simulink model "gm_HDLAWGNGenerator"  (R2021a)
settings: Solver=FixedStepDiscrete  StartTime=0.0  StopTime=StopTime  RelTol=1e-3
InitFcn:
  | whdlexamples.hdlawgn_init
undefined symbols (not defined in the file or in its folder): coefficientsSqrt1, coefficientsSqrt2, SamplingTime, seedsURNG1, seedsURNG2
libraries: hdlsllib x22, simulink x21, dspsrcs4 x1
(part 2 of 2)

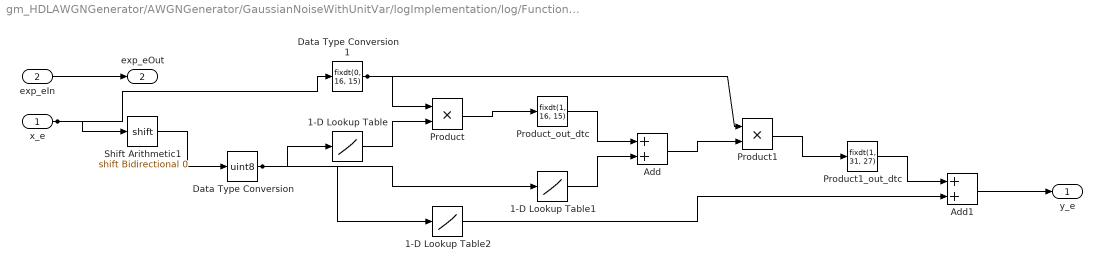
== system gm_HDLAWGNGenerator/AWGNGenerator/GaussianNoiseWithUnitVar/logImplementation/log/FunctionEvaluation ==
  x_e : Inport  OutDataTypeStr=fixdt(0, 49, 48)  PortDimensions=1  SampleTime=1e-06
  exp_eIn : Inport  Port=2  OutDataTypeStr=uint8  PortDimensions=1  SampleTime=1e-06
  1-D Lookup Table : Lookup_n-D  NumberOfTableDimensions=1  BreakpointsForDimension1="fi(\"numerictype\",numerictype(0,8,0),\"fimath\",fimath(\"RoundingMethod\", \"Nearest\",\"OverflowAction\", \"Saturate\",\"ProductMode\",\"FullPrecision\",\"SumMode\",\"FullPrecision\"),\"Value\",\"[0 1 2 3 4 5 6 7 8 9 10 11 12 13 14 15 16 17 18 19 20 21 22 23 24 25 26 27 28 29 30 31 32 33 34 35 36 37 38 39 40 41 42 43 44 45 46 47 48 49 50 51 52 53 54 55 56 57 58 59 60 61 62 63 64 65 66 67 68 69 70 71 72 73 74 75 76 77 78 79 80 81 82 83 84 85 86 87 88 89 90 91 92 93 94 95 96 97 98 99 100 101 102 103 104 105 106 107 108 109 110 111 112 113 114 115 116 117 118 119 120 121 122 123 124 125 126 127 128 129 130 131 132 133 134 135 136 137 138 139 140 141 142 143 144 145 146 147 148 149 150 151 152 153 154 155 156 157 158 159 160 161 162 163 164 165 166 167 168 169 170 171 172 173 174 175 176 177 178 179 180 181 182 183 184 185 186 187 188 189 190 191 192 193 194 195 196 197 198 199 200 201 202 203 204 205 206 207 208 209 210 211 212 213 214 215 216 217 218 219 220 221 222 223 224 225 226 227 228 229 230 231 232 233 234 235 236 237 238 239 240 241 242 243 244 245 246 247 248 249 250 251 252 253 254 255]\")"  Table="reshape(fi(\"numerictype\",numerictype(1,16,15),\"fimath\",fimath(\"RoundingMethod\", \"Floor\",\"OverflowAction\", \"Wrap\",\"ProductMode\",\"FullPrecision\",\"SumMode\",\"FullPrecision\"),\"Value\",\"[-0.498046875;-0.49420166015625;-0.490386962890625;-0.486602783203125;-0.482879638671875;-0.47918701171875;-0.475555419921875;-0.471954345703125;-0.4683837890625;-0.464874267578125;-0.46136474609375;-0.45794677734375;-0.45452880859375;-0.451171875;-0.447845458984375;-0.444549560546875;-0.4412841796875;-0.43804931640625;-0.43487548828125;-0.431732177734375;-0.428619384765625;-0.425537109375;-0.4224853515625;-0.419464111328125;-0.416473388671875;-0.41351318359375;-0.41058349609375;-0.40771484375;-0.40484619140625;-0.402008056640625;-0.399200439453125;-0.39642333984375;-0.393707275390625;-0.3909912109375;-0.3883056640625;-0.3856201171875;-0.38299560546875;-0.380401611328125;-0.3778076171875;-0.375274658203125;-0.37274169921875;-0.3702392578125;-0.367767333984375;-0.36529541015625;-0.362884521484375;-0.3604736328125;-0.35809326171875;-0.355743408203125;-0.3533935546875;-0.351104736328125;-0.34881591796875;-0.3465576171875;-0.34429931640625;-0.342071533203125;-0.339874267578125;-0.33770751953125;-0.335540771484375;-0.333404541015625;-0.331298828125;-0.329193115234375;-0.327117919921875;-0.3250732421875;-0.323028564453125;-0.321014404296875;-0.319000244140625;-0.3170166015625;-0.3150634765625;-0.3131103515625;-0.311187744140625;-0.30926513671875;-0.307373046875;-0.305511474609375;-0.30364990234375;-0.30181884765625;-0.29998779296875;-0.298187255859375;-0.29638671875;-0.29461669921875;-0.2928466796875;-0.291107177734375;-0.289398193359375;-0.287689208984375;-0.285980224609375;-0.2843017578125;-0.282623291015625;-0.280975341796875;-0.279327392578125;-0.2777099609375;-0.276092529296875;-0.274505615234375;-0.272918701171875;-0.2713623046875;-0.269805908203125;-0.26824951171875;-0.2667236328125;-0.265228271484375;-0.263702392578125;-0.262237548828125;-0.2607421875;-0.25927734375;-0.257843017578125;-0.256378173828125;-0.254974365234375;-0.2535400390625;-0.25213623046875;-0.250732421875;-0.249359130859375;-0.24798583984375;-0.24664306640625;-0.24530029296875;-0.24395751953125;-0.24261474609375;-0.241302490234375;-0.240020751953125;-0.23870849609375;-0.2374267578125;-0.23614501953125;-0.234893798828125;-0.233642578125;-0.232391357421875;-0.231170654296875;-0.229949951171875;-0.228729248046875;-0.227508544921875;-0.226318359375;-0.22515869140625;-0.223968505859375;-0.222808837890625;-0.221649169921875;-0.220489501953125;-0.2193603515625;-0.218231201171875;-0.21710205078125;-0.21600341796875;-0.214874267578125;-0.213775634765625;-0.21270751953125;-0.21160888671875;-0.210540771484375;-0.20947265625;-0.20843505859375;-0.2073974609375;-0.20635986328125;-0.205322265625;-0.20428466796875;-0.203277587890625;-0.2022705078125;-0.201263427734375;-0.20025634765625;-0.19927978515625;-0.19830322265625;-0.19732666015625;-0.196380615234375;-0.195404052734375;-0.1944580078125;-0.193511962890625;-0.19256591796875;-0.191650390625;-0.19073486328125;-0.1898193359375;-0.18890380859375;-0.18798828125;-0.187103271484375;-0.186187744140625;-0.185333251953125;-0.1844482421875;-0.183563232421875;-0.182708740234375;-0.181854248046875;-0.180999755859375;-0.180145263671875;-0.179290771484375;-0.178466796875;-0.177642822265625;-0.17681884765625;-0.175994873046875;-0.1751708984375;-0.17437744140625;-0.173553466796875;-0.172760009765625;-0.171966552734375;-0.17120361328125;-0.17041015625;-0.169647216796875;-0.16888427734375;-0.168121337890625;-0.1673583984375;-0.166595458984375;-0.16583251953125;-0.16510009765625;-0.16436767578125;-0.16363525390625;-0.16290283203125;-0.16217041015625;-0.161468505859375;-0.160736083984375;-0.1600341796875;-0.159332275390625;-0.15863037109375;-0.157928466796875;-0.157257080078125;-0.15655517578125;-0.1558837890625;-0.155181884765625;-0.154510498046875;-0.153839111328125;-0.1531982421875;-0.15252685546875;-0.151885986328125;-0.151214599609375;-0.15057373046875;-0.149932861328125;-0.1492919921875;-0.148651123046875;-0.14801025390625;-0.14739990234375;-0.146759033203125;-0.146148681640625;-0.145538330078125;-0.144927978515625 ...(+656 chars)]\"), [256    1])"  InterpMethod=Flat  ExtrapMethod=Clip  DiagnosticForOutOfRangeInput=Error  SampleTime=1e-06  OutDataTypeStr=fixdt(1, 16, 15)  RndMeth=Simplest  InputSameDT=on
  1-D Lookup Table1 : Lookup_n-D  NumberOfTableDimensions=1  BreakpointsForDimension1="fi(\"numerictype\",numerictype(0,8,0),\"fimath\",fimath(\"RoundingMethod\", \"Nearest\",\"OverflowAction\", \"Saturate\",\"ProductMode\",\"FullPrecision\",\"SumMode\",\"FullPrecision\"),\"Value\",\"[0 1 2 3 4 5 6 7 8 9 10 11 12 13 14 15 16 17 18 19 20 21 22 23 24 25 26 27 28 29 30 31 32 33 34 35 36 37 38 39 40 41 42 43 44 45 46 47 48 49 50 51 52 53 54 55 56 57 58 59 60 61 62 63 64 65 66 67 68 69 70 71 72 73 74 75 76 77 78 79 80 81 82 83 84 85 86 87 88 89 90 91 92 93 94 95 96 97 98 99 100 101 102 103 104 105 106 107 108 109 110 111 112 113 114 115 116 117 118 119 120 121 122 123 124 125 126 127 128 129 130 131 132 133 134 135 136 137 138 139 140 141 142 143 144 145 146 147 148 149 150 151 152 153 154 155 156 157 158 159 160 161 162 163 164 165 166 167 168 169 170 171 172 173 174 175 176 177 178 179 180 181 182 183 184 185 186 187 188 189 190 191 192 193 194 195 196 197 198 199 200 201 202 203 204 205 206 207 208 209 210 211 212 213 214 215 216 217 218 219 220 221 222 223 224 225 226 227 228 229 230 231 232 233 234 235 236 237 238 239 240 241 242 243 244 245 246 247 248 249 250 251 252 253 254 255]\")"  Table="reshape(fi(\"numerictype\",numerictype(1,16,14),\"fimath\",fimath(\"RoundingMethod\", \"Floor\",\"OverflowAction\", \"Wrap\",\"ProductMode\",\"FullPrecision\",\"SumMode\",\"FullPrecision\"),\"Value\",\"[1.99609375;1.98834228515625;1.98065185546875;1.9730224609375;1.9654541015625;1.95794677734375;1.95050048828125;1.94305419921875;1.93572998046875;1.928466796875;1.92120361328125;1.91400146484375;1.90692138671875;1.89984130859375;1.892822265625;1.88580322265625;1.87890625;1.87200927734375;1.865234375;1.85845947265625;1.85174560546875;1.84503173828125;1.83843994140625;1.83184814453125;1.8253173828125;1.81884765625;1.8123779296875;1.80596923828125;1.79962158203125;1.7933349609375;1.787109375;1.7808837890625;1.77471923828125;1.7685546875;1.762451171875;1.75640869140625;1.75042724609375;1.74444580078125;1.738525390625;1.732666015625;1.726806640625;1.72100830078125;1.71527099609375;1.70953369140625;1.703857421875;1.69818115234375;1.69256591796875;1.68701171875;1.68145751953125;1.67596435546875;1.67047119140625;1.6650390625;1.65966796875;1.654296875;1.64892578125;1.6436767578125;1.638427734375;1.6331787109375;1.62799072265625;1.622802734375;1.61767578125;1.61260986328125;1.6075439453125;1.60247802734375;1.5975341796875;1.592529296875;1.58758544921875;1.58270263671875;1.57781982421875;1.57293701171875;1.56817626953125;1.5633544921875;1.55859375;1.55389404296875;1.5491943359375;1.54449462890625;1.53985595703125;1.53521728515625;1.5306396484375;1.52606201171875;1.52154541015625;1.51702880859375;1.5125732421875;1.50811767578125;1.503662109375;1.499267578125;1.494873046875;1.49053955078125;1.4862060546875;1.48193359375;1.4776611328125;1.473388671875;1.46917724609375;1.4649658203125;1.46075439453125;1.45660400390625;1.45245361328125;1.4483642578125;1.44427490234375;1.44024658203125;1.4361572265625;1.43218994140625;1.42816162109375;1.4241943359375;1.42022705078125;1.41632080078125;1.41241455078125;1.40850830078125;1.4046630859375;1.40081787109375;1.39697265625;1.3931884765625;1.389404296875;1.38568115234375;1.38189697265625;1.378173828125;1.37451171875;1.37078857421875;1.36712646484375;1.363525390625;1.35992431640625;1.35626220703125;1.35272216796875;1.34912109375;1.3455810546875;1.342041015625;1.33856201171875;1.3350830078125;1.33160400390625;1.328125;1.32470703125;1.3212890625;1.31787109375;1.31451416015625;1.3111572265625;1.30780029296875;1.304443359375;1.3011474609375;1.2978515625;1.2945556640625;1.29132080078125;1.28802490234375;1.2847900390625;1.2816162109375;1.27838134765625;1.27520751953125;1.27203369140625;1.2689208984375;1.2657470703125;1.26263427734375;1.259521484375;1.2564697265625;1.25335693359375;1.25030517578125;1.24725341796875;1.24420166015625;1.2412109375;1.23822021484375;1.2352294921875;1.23223876953125;1.22930908203125;1.226318359375;1.223388671875;1.22052001953125;1.21759033203125;1.2147216796875;1.21185302734375;1.208984375;1.20611572265625;1.20330810546875;1.200439453125;1.1976318359375;1.19488525390625;1.19207763671875;1.1893310546875;1.18658447265625;1.183837890625;1.18109130859375;1.1783447265625;1.1756591796875;1.1729736328125;1.1702880859375;1.1676025390625;1.16497802734375;1.16229248046875;1.15966796875;1.15704345703125;1.15447998046875;1.15185546875;1.1492919921875;1.14666748046875;1.1441650390625;1.1416015625;1.1390380859375;1.13653564453125;1.13397216796875;1.1314697265625;1.12896728515625;1.12652587890625;1.1240234375;1.12158203125;1.119140625;1.11669921875;1.1142578125;1.11181640625;1.10943603515625;1.1070556640625;1.1046142578125;1.10223388671875;1.09991455078125;1.0975341796875;1.09521484375;1.09283447265625;1.09051513671875;1.08819580078125;1.08587646484375;1.0836181640625;1.081298828125;1.07904052734375;1.0767822265625;1.07452392578125;1.072265625;1.07000732421875;1.0677490234375;1.0655517578125;1.0633544921875;1.0611572265625;1.0589599609375;1.0567626953125;1.0545654296875;1.05242919921875;1.05023193359375;1.048095703125;1.04595947265625;1.0438232421875;1.04168701171875;1.03961181640625;1.0374755859375;1.035400390625;1.0333251953125;1.03118896484375;1.0291748046875;1.027099609375;1.0250244140625;1.02294921875;1.02093505859375;1.0189208984375;1.01690673828125;1.014892578125;1.01287841796875;1.0108642578125;1.00885009765625;1.00689697265625;1.0048828125;1.0029296875;1.0009765625]\"), [256    1])"  InterpMethod=Flat  ExtrapMethod=Clip  DiagnosticForOutOfRangeInput=Error  SampleTime=1e-06  OutDataTypeStr=fixdt(1, 16, 14)  RndMeth=Simplest  InputSameDT=on
  1-D Lookup Table2 : Lookup_n-D  NumberOfTableDimensions=1  BreakpointsForDimension1="fi(\"numerictype\",numerictype(0,8,0),\"fimath\",fimath(\"RoundingMethod\", \"Nearest\",\"OverflowAction\", \"Saturate\",\"ProductMode\",\"FullPrecision\",\"SumMode\",\"FullPrecision\"),\"Value\",\"[0 1 2 3 4 5 6 7 8 9 10 11 12 13 14 15 16 17 18 19 20 21 22 23 24 25 26 27 28 29 30 31 32 33 34 35 36 37 38 39 40 41 42 43 44 45 46 47 48 49 50 51 52 53 54 55 56 57 58 59 60 61 62 63 64 65 66 67 68 69 70 71 72 73 74 75 76 77 78 79 80 81 82 83 84 85 86 87 88 89 90 91 92 93 94 95 96 97 98 99 100 101 102 103 104 105 106 107 108 109 110 111 112 113 114 115 116 117 118 119 120 121 122 123 124 125 126 127 128 129 130 131 132 133 134 135 136 137 138 139 140 141 142 143 144 145 146 147 148 149 150 151 152 153 154 155 156 157 158 159 160 161 162 163 164 165 166 167 168 169 170 171 172 173 174 175 176 177 178 179 180 181 182 183 184 185 186 187 188 189 190 191 192 193 194 195 196 197 198 199 200 201 202 203 204 205 206 207 208 209 210 211 212 213 214 215 216 217 218 219 220 221 222 223 224 225 226 227 228 229 230 231 232 233 234 235 236 237 238 239 240 241 242 243 244 245 246 247 248 249 250 251 252 253 254 255]\")"  Table="reshape(fi(\"numerictype\",numerictype(1,32,30),\"fimath\",fimath(\"RoundingMethod\", \"Floor\",\"OverflowAction\", \"Wrap\",\"ProductMode\",\"FullPrecision\",\"SumMode\",\"FullPrecision\"),\"Value\",\"[-1.4980503544211387634;-1.494159286841750145;-1.4902833001688122749;-1.4864222798496484756;-1.4825761094689369202;-1.4787446754053235054;-1.4749278659000992775;-1.471125568263232708;-1.4673376735299825668;-1.4635640727356076241;-1.4598046587780117989;-1.4560593254864215851;-1.4523279676213860512;-1.4486104799434542656;-1.4449067618697881699;-1.4412167100235819817;-1.4375402247533202171;-1.433877207338809967;-1.4302275581285357475;-1.4265911802649497986;-1.4229679778218269348;-1.4193578558042645454;-1.4157607201486825943;-1.4121764777228236198;-1.4086050363257527351;-1.4050463037565350533;-1.4015001915395259857;-1.3979666102677583694;-1.3944454705342650414;-1.3909366857260465622;-1.3874401701614260674;-1.3839558372274041176;-1.3804836031049489975;-1.3770233830437064171;-1.3735750950872898102;-1.3701386572793126106;-1.3667139885947108269;-1.3633010080084204674;-1.3598996354267001152;-1.3565097935497760773;-1.3531314041465520859;-1.3497643899172544479;-1.3464086735621094704;-1.3430641815066337585;-1.339730837382376194;-1.3364085676148533821;-1.3330972986295819283;-1.329796958714723587;-1.3265074742957949638;-1.3232287755236029625;-1.3199607916176319122;-1.3167034527286887169;-1.3134566890075802803;-1.3102204333990812302;-1.3069946169853210449;-1.3037791736423969269;-1.3005740363150835037;-1.2973791379481554031;-1.2941944152116775513;-1.291019802913069725;-1.287855236791074276;-1.2847006535157561302;-1.2815559906885027885;-1.2784211849793791771;-1.2752961767837405205;-1.2721809027716517448;-1.2690753042697906494;-1.2659793198108673096;-1.2628928916528820992;-1.2598159601911902428;-1.2567484676837921143;-1.2536903554573655128;-1.250641566701233387;-1.2476020446047186852;-1.2445717332884669304;-1.2415505778044462204;-1.2385385213419795036;-1.2355355098843574524;-1.2325414903461933136;-1.2295564077794551849;-1.2265802100300788879;-1.2236128430813550949;-1.220654255710542202;-1.2177043957635760307;-1.2147632120177149773;-1.2118306532502174377;-1.2089066701009869576;-1.2059912104159593582;-1.2030842266976833344;-1.2001856686547398567;-1.1972954887896776199;-1.1944136368110775948;-1.191540067084133625;-1.1886747311800718307;-1.1858175806701183319;-1.1829685717821121216;-1.1801276560872793198;-1.1772947879508137703;-1.1744699226692318916;-1.1716530146077275276;-1.1688440199941396713;-1.166042892262339592;-1.1632495904341340065;-1.1604640688747167587;-1.1576862847432494164;-1.1549161951988935471;-1.1521537583321332932;-1.1493989313021302223;-1.1466516721993684769;-1.1439119409769773483;-1.1411796938627958298;-1.138454892672598362;-1.1357374954968690872;-1.1330274622887372971;-1.1303247539326548576;-1.1276293303817510605;-1.1249411534518003464;-1.1222601821646094322;-1.119586380198597908;-1.1169197075068950653;-1.1142601277679204941;-1.1116076027974486351;-1.1089620944112539291;-1.1063235672190785408;-1.1036919821053743362;-1.1010673055425286293;-1.0984494993463158607;-1.0958385281264781952;-1.0932343564927577972;-1.0906369481235742569;-1.088046269491314888;-1.0854622852057218552;-1.0828849608078598976;-1.0803142618387937546;-1.0777501547709107399;-1.0751926051452755928;-1.0726415794342756271;-1.0700970450416207314;-1.0675589693710207939;-1.0650273198261857033;-1.0625020619481801987;-1.0599831659346818924;-1.0574705982580780983;-1.0549643281847238541;-1.0524643240496516228;-1.0499705532565712929;-1.0474829869344830513;-1.0450015924870967865;-1.0425263410434126854;-1.0400572009384632111;-1.0375941423699259758;-1.0351371355354785919;-1.0326861506327986717;-1.0302411587908864021;-1.0278021302074193954;-1.0253690360113978386;-1.0229418473318219185;-1.0205205362290143967;-1.0181050729006528854;-1.0156954303383827209;-1.0132915796712040901;-1.0108934938907623291;-1.008501145988702774;-1.0061145070940256119;-1.0037335511296987534;-1.00135825015604496;-0.99898857809603214264;-0.99662450794130563736;-0.99426601361483335495;-0.99191306903958320618;-0.98956564720720052719;-0.98722372297197580338;-0.9848872702568769455;-0.98255626484751701355 ...(+1957 chars)]\"), [256    1])"  InterpMethod=Flat  ExtrapMethod=Clip  DiagnosticForOutOfRangeInput=Error  SampleTime=1e-06  OutDataTypeStr=fixdt(1, 32, 30)  RndMeth=Simplest  InputSameDT=on
  Add : Sum  AccumDataTypeStr=fixdt(1, 18, 15)  OutDataTypeStr=fixdt(1, 16, 14)  SampleTime=1e-06
  Add1 : Sum  AccumDataTypeStr=fixdt(1, 35, 30)  OutDataTypeStr=fixdt(1, 31, 27)  SampleTime=1e-06
  Data Type Conversion : DataTypeConversion  OutDataTypeStr=uint8  SampleTime=1e-06
  Data Type Conversion1 : DataTypeConversion  OutDataTypeStr=fixdt(0, 16, 15)  SampleTime=1e-06
  Product : Product  Inputs=**  OutDataTypeStr=fixdt(1, 32, 30)  SampleTime=1e-06
  Product1 : Product  Inputs=**  OutDataTypeStr=fixdt(1, 32, 29)  SampleTime=1e-06
  Product1_out_dtc : DataTypeConversion  OutDataTypeStr=fixdt(1, 31, 27)  SampleTime=1e-06
  Product_out_dtc : DataTypeConversion  OutDataTypeStr=fixdt(1, 16, 15)  SampleTime=1e-06
  Shift Arithmetic1 : ArithShift  BinPtShiftNumber=double(8)
  y_e : Outport  SampleTime=1e-06
  exp_eOut : Outport  Port=2  SampleTime=1e-06
  wires:
  x_e/1 -> Shift Arithmetic1/1, Data Type Conversion1/1
  exp_eIn/1 -> exp_eOut/1
  1-D Lookup Table/1 -> Product/2
  1-D Lookup Table1/1 -> Add/2
  1-D Lookup Table2/1 -> Add1/2
  Add/1 -> Product1/2
  Add1/1 -> y_e/1
  Data Type Conversion/1 -> 1-D Lookup Table2/1, 1-D Lookup Table1/1, 1-D Lookup Table/1
  Data Type Conversion1/1 -> Product1/1, Product/1
  Product_out_dtc/1 -> Add/1
  Product1_out_dtc/1 -> Add1/1
  Shift Arithmetic1/1 -> Data Type Conversion/1
  Product/1 -> Product_out_dtc/1
  Product1/1 -> Product1_out_dtc/1

== system gm_HDLAWGNGenerator/AWGNGenerator/GaussianNoiseWithUnitVar/logImplementation/log/RangeReconstruction ==
  y_e : Inport  OutDataTypeStr=fixdt(1, 31, 27)  PortDimensions=1  SampleTime=1e-06
  exp_e : Inport  Port=2  OutDataTypeStr=uint8  PortDimensions=1  SampleTime=1e-06
  Add1 : Sum  Inputs=+-  AccumDataTypeStr=fixdt(1, 36, 28)  OutDataTypeStr=fixdt(0, 31, 24)  SampleTime=1e-06
  Bit Shift : hdlsllib/Logic and Bit Operations/Bit Shift  mode=Shift Left Logical  N=double(1)
  Constant : Constant  Value=0.69314718060195446014404296875  OutDataTypeStr=fixdt(1, 33, 32)  SampleTime=1e-06
  Product : Product  Inputs=**  OutDataTypeStr=fixdt(1, 41, 32)  SampleTime=1e-06
  Product_out_dtc : DataTypeConversion  OutDataTypeStr=fixdt(1, 35, 28)  SampleTime=1e-06
  e : Outport  SampleTime=1e-06
  wires:
  y_e/1 -> Add1/2
  exp_e/1 -> Product/1
  Add1/1 -> Bit Shift/1
  Bit Shift/1 -> e/1
  Constant/1 -> Product/2
  Product_out_dtc/1 -> Add1/1
  Product/1 -> Product_out_dtc/1

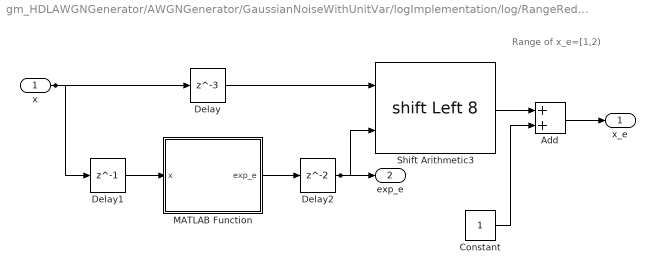
== system gm_HDLAWGNGenerator/AWGNGenerator/GaussianNoiseWithUnitVar/logImplementation/log/RangeReduction ==
  note: Range of x_e=[1,2)
  x : Inport  OutDataTypeStr=fixdt(0, 48, 48)  PortDimensions=1  SampleTime=1e-06
  Add : Sum  OutDataTypeStr=fixdt(0,49,48)
  Constant : Constant  OutDataTypeStr=uint8  SampleTime=-1
  Delay : Delay  DelayLength=3
  Delay1 : Delay  DelayLength=1
  Delay2 : Delay
  MATLAB Function : Subsystem
  Shift Arithmetic3 : ArithShift  BitShiftNumberSource=Input port  BitShiftNumber=8  BitShiftDirection=Left
      settings: InputPortMap=u0,p1
  x_e : Outport  SampleTime=1e-06
  exp_e : Outport  Port=2  SampleTime=1e-06  VectorParamsAs1DForOutWhenUnconnected=off
  wires:
  x/1 -> Delay1/1, Delay/1
  Add/1 -> x_e/1
  Constant/1 -> Add/2
  Delay/1 -> Shift Arithmetic3/1
  Delay1/1 -> MATLAB Function/1(x)
  Delay2/1 -> Shift Arithmetic3/2, exp_e/1
  MATLAB Function/1(exp_e) -> Delay2/1
  Shift Arithmetic3/1 -> Add/1

== system gm_HDLAWGNGenerator/AWGNGenerator/GaussianNoiseWithUnitVar/SqrtImplementation/SqrtEval/RangeReduction/MATLAB Function ==
  x : Inport  OutDataTypeStr=fixdt(0, 31, 24)  PortDimensions=1  SampleTime=1e-06
  MATLAB Function : MATLAB Function  TreatAsAtomicUnit=on
  exp_f : Outport  SampleTime=1e-06  VectorParamsAs1DForOutWhenUnconnected=off
  wires:
  x/1 -> MATLAB Function/1(x)
  MATLAB Function/1(exp_f) -> exp_f/1

== system gm_HDLAWGNGenerator/AWGNGenerator/GaussianNoiseWithUnitVar/logImplementation/log/RangeReduction/MATLAB Function ==
  x : Inport  OutDataTypeStr=fixdt(0, 48, 48)  PortDimensions=1  SampleTime=1e-06
  MATLAB Function : MATLAB Function  TreatAsAtomicUnit=on
  exp_e : Outport  SampleTime=1e-06  VectorParamsAs1DForOutWhenUnconnected=off
  wires:
  x/1 -> MATLAB Function/1(x)
  MATLAB Function/1(exp_e) -> exp_e/1

== matlab function gm_HDLAWGNGenerator/AWGNGenerator/GaussianNoiseWithUnitVar/logImplementation/log/RangeReduction/MATLAB Function/MATLAB Function ==
  data: x input; exp_e output
function exp_e=leadingZeroDetector(x)
temp = 0;
flag=1.0e+14 *[0.000000000000020
   0.000000000000040
   0.000000000000080
   0.000000000000160
   0.000000000000320
   0.000000000000640
   0.000000000001280
   0.000000000002560
   0.000000000005120
   0.000000000010240
   0.000000000020480
   0.000000000040960
   0.000000000081920
   0.000000000163840
   0.000000000327680
   0.000000000655360
   0.000000001310720
   0.000000002621440
   0.000000005242880
   0.000000010485760
   0.000000020971520
   0.000000041943040
   0.000000083886080
   0.000000167772160
   0.000000335544320
   0.000000671088640
   0.000001342177280
   0.000002684354560
   0.000005368709120
   0.000010737418240
   0.000021474836480
   0.000042949672960
   0.000085899345920
   0.000171798691840
   0.000343597383680
   0.000687194767360
   0.001374389534720
   0.002748779069440
   0.005497558138880
   0.010995116277760
   0.021990232555520
   0.043980465111040
   0.087960930222080
   0.175921860444160
   0.351843720888320
   0.703687441776640
   1.407374883553280
   2.814749767106560];

% else
%     while( )
%         temp = temp+1;
%         flag()=flag()*2;
%     end
% end
% 
% end
if(x == 0)
     temp = 49;
elseif (x*flag(1)>1)
        temp=1;
elseif (x*flag(2)>1)
        temp=2;
elseif (x*flag(3)>1)
        temp=3;
elseif (x*flag(4)>1)
        temp=4;
elseif (x*flag(5)>1)
        temp=5;
elseif (x*flag(6)>1)
        temp=6;
elseif (x*flag(7)>1)
        temp=7;
elseif (x*flag(8)>1)
        temp=8;
elseif (x*flag(9)>1)
        temp=9;
elseif (x*flag(10)>1)
        temp=10;
elseif (x*flag(11)>1)
        temp=11;
elseif (x*flag(12)>1)
        temp=12;
elseif (x*flag(13)>1)
        temp=13;
elseif (x*flag(14)>1)
        temp=14;
elseif (x*flag(15)>1)
        temp=15;
elseif (x*flag(16)>1)
        temp=16;
elseif (x*flag(17)>1)
        temp=17;
elseif (x*flag(18)>1)
        temp=18;
elseif (x*flag(19)>1)
        temp=19;
elseif (x*flag(20)>1)
        temp=20;
elseif (x*flag(21)>1)
        temp=21;
elseif (x*flag(22)>1)
        temp=22;
elseif (x*flag(23)>1)
        temp=23;
elseif (x*flag(24)>1)
        temp=24;
elseif (x*flag(25)>1)
        temp=25;
elseif (x*flag(26)>1)
        temp=26;
elseif (x*flag(27)>1)
        temp=27;
elseif (x*flag(28)>1)
        temp=28;
elseif (x*flag(29)>1)
        temp=29;
elseif (x*flag(30)>1)
        temp=30;
elseif (x*flag(31)>1)
        temp=31;
elseif (x*flag(32)>1)
        temp=32;
elseif (x*flag(33)>1)
        temp=33;
elseif (x*flag(34)>1)
        temp=34;
elseif (x*flag(35)>1)
        temp=35;
elseif (x*flag(36)>1)
        temp=36;
elseif (x*flag(37)>1)
        temp=37;
elseif (x*flag(38)>1)
        temp=8;
elseif (x*flag(39)>1)
        temp=39;
elseif (x*flag(40)>1)
        temp=40;
elseif (x*flag(41)>1)
        temp=41;
elseif (x*flag(42)>1)
        temp=42;
elseif (x*flag(43)>1)
        temp=43;
elseif (x*flag(44)>1)
        temp=44;
elseif (x*flag(45)>1)
        temp=45;
elseif (x*flag(46)>1)
        temp=46;
elseif (x*flag(47)>1)
        temp=47; 
elseif (x*flag(48)>1)
        temp=48; 
end        
exp_e=uint8(temp);

== matlab function gm_HDLAWGNGenerator/AWGNGenerator/GaussianNoiseWithUnitVar/SqrtImplementation/SqrtEval/RangeReduction/MATLAB Function/MATLAB Function ==
  data: x input; exp_f output
function exp_f=leadingZeroDetector(x)
%exp_e=31-length(dec2bin(x));
x=fi(x,0,38,31);
x = x/2^(6);
temp = 0;
flag=1.0e+09 *[

   0.000000002000000
   0.000000004000000
   0.000000008000000
   0.000000016000000
   0.000000032000000
   0.000000064000000
   0.000000128000000
   0.000000256000000
   0.000000512000000
   0.000001024000000
   0.000002048000000
   0.000004096000000
   0.000008192000000
   0.000016384000000
   0.000032768000000
   0.000065536000000
   0.000131072000000
   0.000262144000000
   0.000524288000000
   0.001048576000000
   0.002097152000000
   0.004194304000000
   0.008388608000000
   0.016777216000000
   0.033554432000000
   0.067108864000000
   0.134217728000000
   0.268435456000000
   0.536870912000000
   1.073741824000000
   2.147483648000000];

% else
%     while( )
%         temp = temp+1;
%         flag()=flag()*2;
%     end
% end
% 
% end
if(x == 0)
     temp = 31;
elseif (x*flag(1)>1)
        temp=1;
elseif (x*flag(2)>1)
        temp=2;
elseif (x*flag(3)>1)
        temp=3;
elseif (x*flag(4)>1)
        temp=4;
elseif (x*flag(5)>1)
        temp=5;
elseif (x*flag(6)>1)
        temp=6;
elseif (x*flag(7)>1)
        temp=7;
elseif (x*flag(8)>1)
        temp=8;
elseif (x*flag(9)>1)
        temp=9;
elseif (x*flag(10)>1)
        temp=10;
elseif (x*flag(11)>1)
        temp=11;
elseif (x*flag(12)>1)
        temp=12;
elseif (x*flag(13)>1)
        temp=13;
elseif (x*flag(14)>1)
        temp=14;
elseif (x*flag(15)>1)
        temp=15;
elseif (x*flag(16)>1)
        temp=16;
elseif (x*flag(17)>1)
        temp=17;
elseif (x*flag(18)>1)
        temp=18;
elseif (x*flag(19)>1)
        temp=19;
elseif (x*flag(20)>1)
        temp=20;
elseif (x*flag(21)>1)
        temp=21;
elseif (x*flag(22)>1)
        temp=22;
elseif (x*flag(23)>1)
        temp=23;
elseif (x*flag(24)>1)
        temp=24;
elseif (x*flag(25)>1)
        temp=25;
elseif (x*flag(26)>1)
        temp=26;
elseif (x*flag(27)>1)
        temp=27;
elseif (x*flag(28)>1)
        temp=28;
elseif (x*flag(29)>1)
        temp=29;
elseif (x*flag(30)>1)
        temp=30;              
end        
exp_f=uint8(temp);
